simulink model "examen_Simulacion_20_12_2019"  (R2024a)
settings: Solver=VariableStepAuto  StartTime=0.0  StopTime=50  RelTol=1e-3
values from neighbouring files (symbols this model uses):
  a_og = 1.697    [examen_20_12_2019.m]
  b_og = 1    [examen_20_12_2019.m]
  h = (2*pi)/(20*Wn)    [examen_20_12_2019.m]
  Mp = 14.77/100    (= 0.1477)    [examen_20_12_2019.m]
undefined symbols (not defined in the file or in its folder): den, K_rlocfind, National_Instruments, num, PCI
libraries: sldrtlib x2
settings Model: Creator=david  LastModifiedBy=david

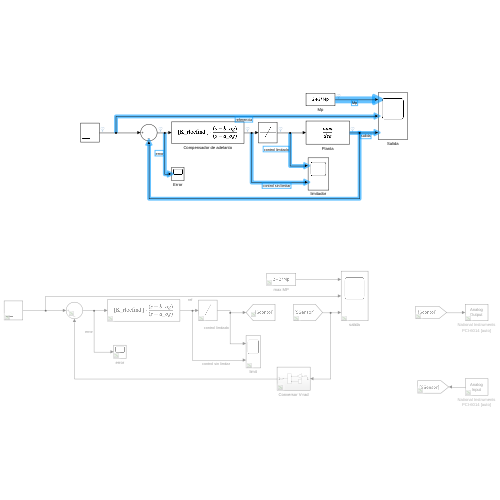
[thumbnail: Simulink's stored preview of the top-level diagram]
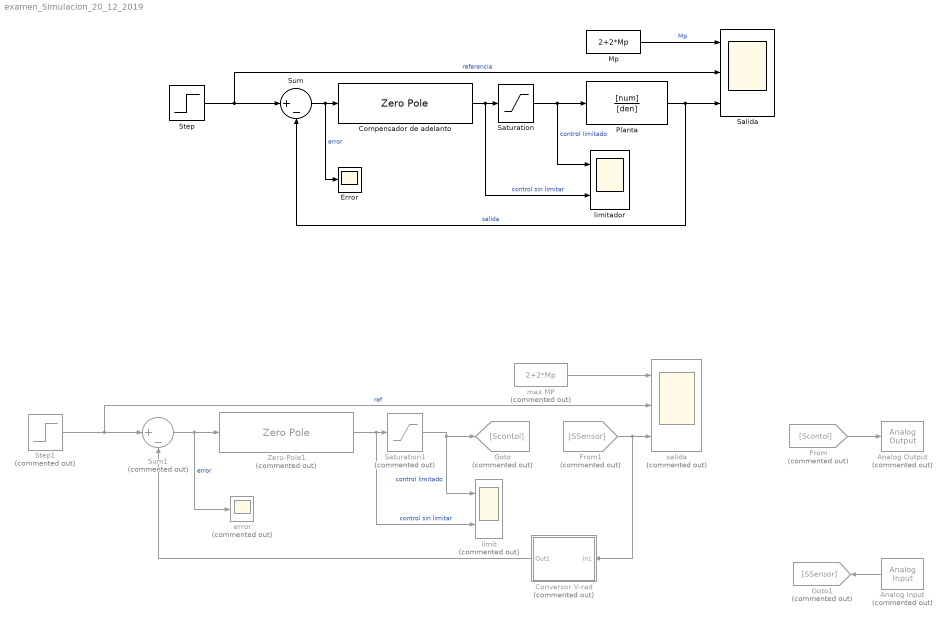
== system examen_Simulacion_20_12_2019 ==
  Analog Input : sldrtlib/Analog Input  Commented=on  SampleTime=h  MaxMissedTicks=10  ShowMissedTicks=off  YieldWhenWaiting=off  DrvName=National_Instruments/PCI-6014  DrvAddress=4294967295  DrvOptions=[0 0 0 0 0 0]  Channels=3  RangeMode=1  VoltRange=1  DataType=1
      settings: AttributesFormatString=National Instruments\nPCI-6014 [auto]
  Analog Output : sldrtlib/Analog Output  Commented=on  SampleTime=h  MaxMissedTicks=10  ShowMissedTicks=off  YieldWhenWaiting=off  DrvName=National_Instruments/PCI-6014  DrvAddress=4294967295  DrvOptions=[0 0 0 0 0 0]  Channels=3  RangeMode=1  VoltRange=1  InitialValue=0  FinalValue=0
      settings: AttributesFormatString=National Instruments\nPCI-6014 [auto]
  Compensador de adelanto : ZeroPole  Zeros=[-b_og]  Poles=[-a_og]  Gain=[K_rlocfind]
  Conversor V-rad : Subsystem  Commented=on
  Error : Scope
  From : From  Commented=on  GotoTag=Scontol
  From1 : From  Commented=on  GotoTag=SSensor
  Goto : Goto  Commented=on  GotoTag=Scontol
  Goto1 : Goto  Commented=on  GotoTag=SSensor
  Mp : Constant  Value=2+2*Mp
  Planta : TransferFcn  Numerator=[num]  Denominator=[den]
  Salida : Scope  NumInputPorts=3
  Saturation : Saturate  UpperLimit=8  LowerLimit=-8
  Saturation1 : Saturate  Commented=on  UpperLimit=8  LowerLimit=-8
  Step : Step  Time=0.5  After=2  SampleTime=h
  Step1 : Step  Commented=on  Time=0.5  After=2  SampleTime=h
  Sum : Sum  Inputs=|+-
  Sum1 : Sum  Commented=on  Inputs=|+-
  Zero-Pole1 : ZeroPole  Commented=on  Zeros=[-b_og]  Poles=[-a_og]  Gain=[K_rlocfind]
  error : Scope  Commented=on
  limit : Scope  Commented=on  NumInputPorts=2
  limitador : Scope  NumInputPorts=2
  max MP : Constant  Commented=on  Value=2+2*Mp
  salida : Scope  Commented=on  NumInputPorts=3
  wires:
  Compensador de adelanto/1 -> limitador/2, Saturation/1  "control sin limitar"
  Step/1 -> Sum/1, Salida/2  "referencia"
  Saturation/1 -> limitador/1, Planta/1  "control limitado"
  Planta/1 -> Sum/2, Salida/3  "salida"
  Mp/1 -> Salida/1  "Mp"
  Step1/1 -> Sum1/1, salida/2  "ref"
  Sum1/1 -> Zero-Pole1/1, error/1  "error"
  Zero-Pole1/1 -> limit/2, Saturation1/1  "control sin limitar"
  max MP/1 -> salida/1
  Saturation1/1 -> Goto/1, limit/1  "control limitado"
  From/1 -> Analog Output/1
  Analog Input/1 -> Goto1/1
  From1/1 -> Conversor V-rad/1(In1), salida/3
  Sum/1 -> Error/1, Compensador de adelanto/1  "error"
  Conversor V-rad/1(Out1) -> Sum1/2

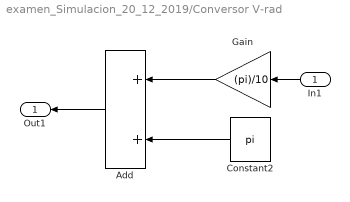
== system examen_Simulacion_20_12_2019/Conversor V-rad ==
  In1 : Inport
  Add : Sum
  Constant2 : Constant  Value=pi
  Gain : Gain  Gain=(pi)/10
  Out1 : Outport
  wires:
  Constant2/1 -> Add/2
  Gain/1 -> Add/1
  Add/1 -> Out1/1
  In1/1 -> Gain/1
